simulink model "Damp"  (R2016b)
settings: Solver=VariableStepAuto  StartTime=0.0  StopTime=100.0  RelTol=1e-3
settings Model: Creator=Administrator  LastModifiedBy=Administrator

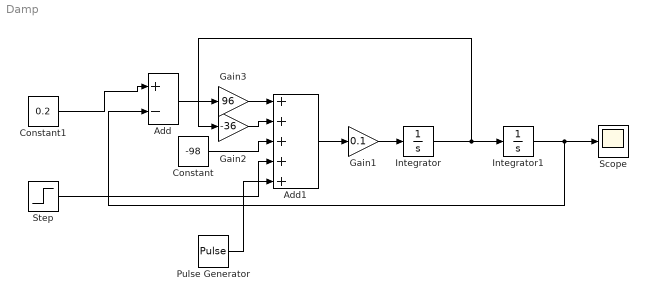
== system Damp ==
  Add : Sum  Inputs=+-
  Add1 : Sum  Inputs=+++++
  Constant : Constant  Value=-98
  Constant1 : Constant  Value=0.2
  Gain1 : Gain  Gain=0.1
  Gain2 : Gain  Gain=-36
  Gain3 : Gain  Gain=96
  Integrator : Integrator
  Integrator1 : Integrator  InitialCondition=0.1
  Pulse Generator : DiscretePulseGenerator  Amplitude=10  Period=10  PulseWidth=5
  Scope : Scope
  Step : Step  After=0  SampleTime=0
  wires:
  Constant1/1 -> Add/1
  Integrator/1 -> Gain2/1, Integrator1/1
  Integrator1/1 -> Add/2, Scope/1
  Add1/1 -> Gain1/1
  Gain1/1 -> Integrator/1
  Add/1 -> Gain3/1
  Gain2/1 -> Add1/2
  Step/1 -> Add1/4
  Constant/1 -> Add1/3
  Gain3/1 -> Add1/1
  Pulse Generator/1 -> Add1/5
